simulink library "orocomplib"  (R2015b)
settings: Solver=ode45  StartTime=0.0  StopTime=10.0  RelTol=1e-3
settings Model: Creator=laurent  LastModifiedBy=admin
settings DataIOCC: SaveFormat=Array  SaveOutput=off  SignalLogging=off  DSMLogging=off  SaveTime=off
settings OptimizationCC: ExpressionDepthLimit=2147483647
settings DebuggingCC: UnderspecifiedInitializationDetection=Classic  MergeDetectMultiDrivingBlocksExec=none  SolverPrmCheckMsg=warning  StateNameClashWarn=warning
settings HardwareCC: ProdBitPerPointer=32  ProdLargestAtomicFloat=None  ProdIntDivRoundTo=Undefined  ProdEndianess=Unspecified  ProdWordSize=32  ProdHWDeviceType=32-bit Generic
settings GRTTargetCC: GeneratePreprocessorConditionals=Disable all
settings ConfigComp: CovModelRefEnable=Off

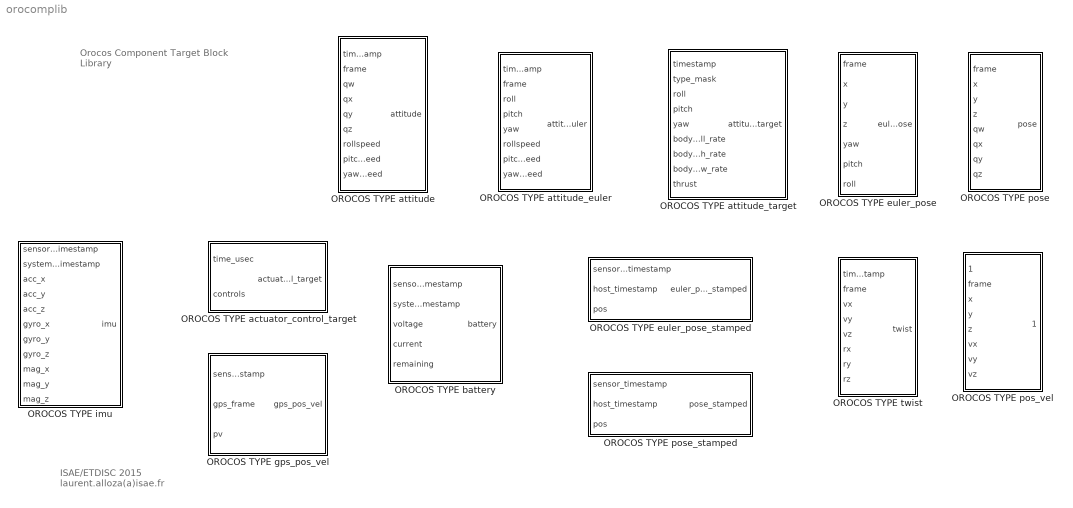
== system orocomplib ==
  note: ISAE/ETDISC 2015
      | laurent.alloza(a)isae.fr
  note: Orocos Component Target
      | Block Library
  OROCOS TYPE battery : Subsystem  InitFcn=|  mask(OROCOS TYPE battery){}
      | if not(exist('battery','var')),
      | load orotypes_isae;
      | end
      mask help: Creates an Orocos Port compatible type.
      settings: MinAlgLoopOccurrences=on  RTWSystemCode=Inline
  OROCOS TYPE imu : Subsystem  InitFcn=|  mask(OROCOS TYPE imu){}
      | if not(exist('imu','var')),
      | load orotypes_isae;
      | end
      mask help: Creates an Orocos Port compatible type.
      settings: MinAlgLoopOccurrences=on  RTWSystemCode=Inline
  OROCOS TYPE actuator_control_target : Subsystem  InitFcn=|  mask(OROCOS TYPE actuator_control_target){}
      | if not(exist('actuator_control_target','var')),
      | load orotypes_isae;
      | end
      mask help: Creates an Orocos Port compatible type.
      settings: MinAlgLoopOccurrences=on  RTWSystemCode=Inline
  OROCOS TYPE attitude : Subsystem  InitFcn=|  mask(OROCOS TYPE attitude){}
      | if not(exist('attitude','var')),
      | load orotypes_isae;
      | end
      mask help: Creates an Orocos Port compatible type.
      settings: MinAlgLoopOccurrences=on  RTWSystemCode=Inline
  OROCOS TYPE attitude_euler : Subsystem  InitFcn=|  mask(OROCOS TYPE attitude_euler){}
      | if not(exist('attitude_euler','var')),
      | load orotypes_isae;
      | end
      mask help: Creates an Orocos Port compatible type.
      settings: MinAlgLoopOccurrences=on  RTWSystemCode=Inline
  OROCOS TYPE attitude_target : Subsystem  InitFcn=|  mask(OROCOS TYPE attitude_target){}
      | if not(exist('attitude_target','var')),
      | load orotypes_isae;
      | end
      mask help: Creates an Orocos Port compatible type.
      settings: MinAlgLoopOccurrences=on  RTWSystemCode=Inline
  OROCOS TYPE euler_pose : Subsystem  InitFcn=|  mask(OROCOS TYPE euler_pose){}
      | if not(exist('euler_pose','var')),
      | load orotypes_isae;
      | end
      mask help: Creates an Orocos Port compatible type.
      settings: MinAlgLoopOccurrences=on  RTWSystemCode=Inline
  OROCOS TYPE euler_pose_stamped : Subsystem  InitFcn=|  mask(OROCOS TYPE euler_pose_stamped){}
      | if not(exist('euler_pose_stamped','var')),
      | load orotypes_isae;
      | end
      mask help: Creates an Orocos Port compatible type.
      settings: MinAlgLoopOccurrences=on  RTWSystemCode=Inline
  OROCOS TYPE gps_pos_vel : Subsystem  InitFcn=|  mask(OROCOS TYPE gps_pos_vel){}
      | if not(exist('gps_pos_vel','var')),
      | load orotypes_isae;
      | end
      mask help: Creates an Orocos Port compatible type.
      settings: MinAlgLoopOccurrences=on  RTWSystemCode=Inline
  OROCOS TYPE pos_vel : Subsystem  InitFcn=|  mask(OROCOS TYPE pos_vel){}
      | if not(exist('pos_vel','var')),
      | load orotypes_isae;
      | end
      mask help: Creates an Orocos Port compatible type.
      settings: MinAlgLoopOccurrences=on  RTWSystemCode=Inline
  OROCOS TYPE pose : Subsystem  InitFcn=|  mask(OROCOS TYPE pose){}
      | if not(exist('pose','var')),
      | load orotypes_isae;
      | end
      mask help: Creates an Orocos Port compatible type.
      settings: MinAlgLoopOccurrences=on  RTWSystemCode=Inline
  OROCOS TYPE pose_stamped : Subsystem  InitFcn=|  mask(OROCOS TYPE pose_stamped){}
      | if not(exist('pose_stamped','var')),
      | load orotypes_isae;
      | end
      mask help: Creates an Orocos Port compatible type.
      settings: MinAlgLoopOccurrences=on  RTWSystemCode=Inline
  OROCOS TYPE twist : Subsystem  InitFcn=|  mask(OROCOS TYPE twist){}
      | if not(exist('twist','var')),
      | load orotypes_isae;
      | end
      mask help: Creates an Orocos Port compatible type.
      settings: MinAlgLoopOccurrences=on  RTWSystemCode=Inline

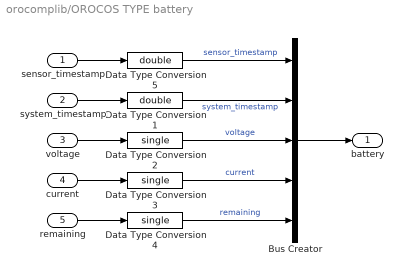
== system orocomplib/OROCOS TYPE battery ==
  sensor_timestamp : Inport  PortDimensions=1
  system_timestamp : Inport  Port=2  PortDimensions=1
  voltage : Inport  Port=3  PortDimensions=1
  current : Inport  Port=4  PortDimensions=1
  remaining : Inport  Port=5  PortDimensions=1
  Bus Creator : BusCreator  Inputs='sensor_timestamp','system_timestamp','voltage','current','remaining'  OutDataTypeStr=Bus: battery  NonVirtualBus=on
  Data Type Conversion1 : DataTypeConversion  OutDataTypeStr=double  RndMeth=Zero  LockScale=on
  Data Type Conversion2 : DataTypeConversion  OutDataTypeStr=single  RndMeth=Zero  LockScale=on
  Data Type Conversion3 : DataTypeConversion  OutDataTypeStr=single  RndMeth=Zero  LockScale=on
  Data Type Conversion4 : DataTypeConversion  OutDataTypeStr=single  RndMeth=Zero  LockScale=on
  Data Type Conversion5 : DataTypeConversion  OutDataTypeStr=double  RndMeth=Zero  LockScale=on
  battery : Outport
  wires:
  system_timestamp/1 -> Data Type Conversion1/1
  Data Type Conversion1/1 -> Bus Creator/2  "system_timestamp"
  Data Type Conversion4/1 -> Bus Creator/5  "remaining"
  remaining/1 -> Data Type Conversion4/1
  Data Type Conversion3/1 -> Bus Creator/4  "current"
  current/1 -> Data Type Conversion3/1
  Data Type Conversion2/1 -> Bus Creator/3  "voltage"
  voltage/1 -> Data Type Conversion2/1
  sensor_timestamp/1 -> Data Type Conversion5/1
  Bus Creator/1 -> battery/1
  Data Type Conversion5/1 -> Bus Creator/1  "sensor_timestamp"

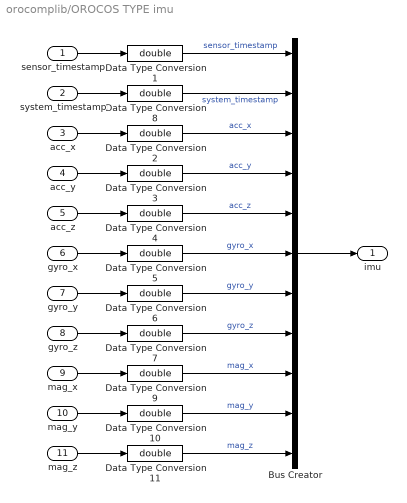
== system orocomplib/OROCOS TYPE imu ==
  sensor_timestamp : Inport  PortDimensions=1
  system_timestamp : Inport  Port=2  PortDimensions=1
  acc_x : Inport  Port=3  PortDimensions=1
  acc_y : Inport  Port=4  PortDimensions=1
  acc_z : Inport  Port=5  PortDimensions=1
  gyro_x : Inport  Port=6  PortDimensions=1
  gyro_y : Inport  Port=7  PortDimensions=1
  gyro_z : Inport  Port=8  PortDimensions=1
  mag_x : Inport  Port=9  PortDimensions=1
  mag_y : Inport  Port=10  PortDimensions=1
  mag_z : Inport  Port=11  PortDimensions=1
  Bus Creator : BusCreator  Inputs=11  OutDataTypeStr=Bus: imu  NonVirtualBus=on
  Data Type Conversion{1..11} (11 alike) : DataTypeConversion  OutDataTypeStr=double  RndMeth=Zero  LockScale=on
  imu : Outport
  wires:
  system_timestamp/1 -> Data Type Conversion8/1
  Data Type Conversion8/1 -> Bus Creator/2  "system_timestamp"
  Data Type Conversion2/1 -> Bus Creator/3  "acc_x"
  acc_x/1 -> Data Type Conversion2/1
  sensor_timestamp/1 -> Data Type Conversion1/1
  Bus Creator/1 -> imu/1
  Data Type Conversion1/1 -> Bus Creator/1  "sensor_timestamp"
  Data Type Conversion3/1 -> Bus Creator/4  "acc_y"
  acc_y/1 -> Data Type Conversion3/1
  Data Type Conversion4/1 -> Bus Creator/5  "acc_z"
  acc_z/1 -> Data Type Conversion4/1
  Data Type Conversion5/1 -> Bus Creator/6  "gyro_x"
  gyro_x/1 -> Data Type Conversion5/1
  Data Type Conversion6/1 -> Bus Creator/7  "gyro_y"
  gyro_y/1 -> Data Type Conversion6/1
  Data Type Conversion7/1 -> Bus Creator/8  "gyro_z"
  gyro_z/1 -> Data Type Conversion7/1
  Data Type Conversion9/1 -> Bus Creator/9  "mag_x"
  mag_x/1 -> Data Type Conversion9/1
  Data Type Conversion10/1 -> Bus Creator/10  "mag_y"
  mag_y/1 -> Data Type Conversion10/1
  Data Type Conversion11/1 -> Bus Creator/11  "mag_z"
  mag_z/1 -> Data Type Conversion11/1

== system orocomplib/OROCOS TYPE actuator_control_target ==
  time_usec : Inport  PortDimensions=1
  controls : Inport  Port=2  PortDimensions=8
  Bus Creator : BusCreator  Inputs=2  OutDataTypeStr=Bus: actuator_control_target  NonVirtualBus=on
  Data Type Conversion1 : DataTypeConversion  OutDataTypeStr=double  RndMeth=Zero  LockScale=on
  Data Type Conversion2 : DataTypeConversion  OutDataTypeStr=single  RndMeth=Zero  LockScale=on
  actuator_control_target : Outport
  wires:
  Data Type Conversion2/1 -> Bus Creator/2  "controls"
  controls/1 -> Data Type Conversion2/1
  time_usec/1 -> Data Type Conversion1/1
  Bus Creator/1 -> actuator_control_target/1
  Data Type Conversion1/1 -> Bus Creator/1  "time_usec"

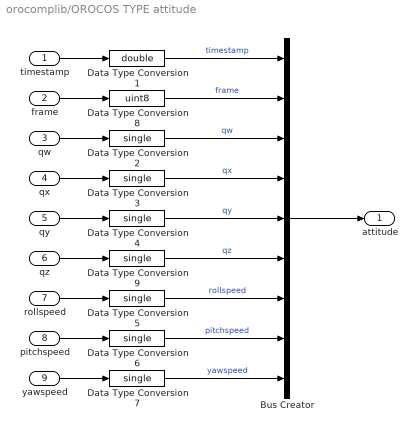
== system orocomplib/OROCOS TYPE attitude ==
  timestamp : Inport  PortDimensions=1
  frame : Inport  Port=2  PortDimensions=1
  qw : Inport  Port=3  PortDimensions=1
  qx : Inport  Port=4  PortDimensions=1
  qy : Inport  Port=5  PortDimensions=1
  qz : Inport  Port=6  PortDimensions=1
  rollspeed : Inport  Port=7  PortDimensions=1
  pitchspeed : Inport  Port=8  PortDimensions=1
  yawspeed : Inport  Port=9  PortDimensions=1
  Bus Creator : BusCreator  Inputs='timestamp','frame','qw','qx','qy','qz','rollspeed','pitchspeed','yawspeed'  OutDataTypeStr=Bus: attitude  NonVirtualBus=on
  Data Type Conversion1 : DataTypeConversion  OutDataTypeStr=double  RndMeth=Zero  LockScale=on
  Data Type Conversion{2..7,9} (7 alike) : DataTypeConversion  OutDataTypeStr=single  RndMeth=Zero  LockScale=on
  Data Type Conversion8 : DataTypeConversion  OutDataTypeStr=uint8  RndMeth=Zero  LockScale=on
  attitude : Outport
  wires:
  qz/1 -> Data Type Conversion9/1
  Data Type Conversion9/1 -> Bus Creator/6  "qz"
  Data Type Conversion1/1 -> Bus Creator/1  "timestamp"
  frame/1 -> Data Type Conversion8/1
  Bus Creator/1 -> attitude/1
  timestamp/1 -> Data Type Conversion1/1
  qw/1 -> Data Type Conversion2/1
  Data Type Conversion2/1 -> Bus Creator/3  "qw"
  qx/1 -> Data Type Conversion3/1
  Data Type Conversion3/1 -> Bus Creator/4  "qx"
  qy/1 -> Data Type Conversion4/1
  Data Type Conversion4/1 -> Bus Creator/5  "qy"
  rollspeed/1 -> Data Type Conversion5/1
  pitchspeed/1 -> Data Type Conversion6/1
  yawspeed/1 -> Data Type Conversion7/1
  Data Type Conversion5/1 -> Bus Creator/7  "rollspeed"
  Data Type Conversion6/1 -> Bus Creator/8  "pitchspeed"
  Data Type Conversion7/1 -> Bus Creator/9  "yawspeed"
  Data Type Conversion8/1 -> Bus Creator/2  "frame"

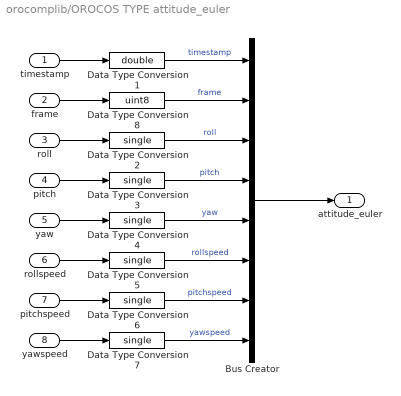
== system orocomplib/OROCOS TYPE attitude_euler ==
  timestamp : Inport  PortDimensions=1
  frame : Inport  Port=2  PortDimensions=1
  roll : Inport  Port=3  PortDimensions=1
  pitch : Inport  Port=4  PortDimensions=1
  yaw : Inport  Port=5  PortDimensions=1
  rollspeed : Inport  Port=6  PortDimensions=1
  pitchspeed : Inport  Port=7  PortDimensions=1
  yawspeed : Inport  Port=8  PortDimensions=1
  Bus Creator : BusCreator  Inputs=8  OutDataTypeStr=Bus: attitude_euler  NonVirtualBus=on
  Data Type Conversion1 : DataTypeConversion  OutDataTypeStr=double  RndMeth=Zero  LockScale=on
  Data Type Conversion{2..7} (6 alike) : DataTypeConversion  OutDataTypeStr=single  RndMeth=Zero  LockScale=on
  Data Type Conversion8 : DataTypeConversion  OutDataTypeStr=uint8  RndMeth=Zero  LockScale=on
  attitude_euler : Outport
  wires:
  Data Type Conversion1/1 -> Bus Creator/1  "timestamp"
  frame/1 -> Data Type Conversion8/1
  Bus Creator/1 -> attitude_euler/1
  timestamp/1 -> Data Type Conversion1/1
  roll/1 -> Data Type Conversion2/1
  Data Type Conversion2/1 -> Bus Creator/3  "roll"
  pitch/1 -> Data Type Conversion3/1
  Data Type Conversion3/1 -> Bus Creator/4  "pitch"
  yaw/1 -> Data Type Conversion4/1
  Data Type Conversion4/1 -> Bus Creator/5  "yaw"
  rollspeed/1 -> Data Type Conversion5/1
  pitchspeed/1 -> Data Type Conversion6/1
  yawspeed/1 -> Data Type Conversion7/1
  Data Type Conversion5/1 -> Bus Creator/6  "rollspeed"
  Data Type Conversion6/1 -> Bus Creator/7  "pitchspeed"
  Data Type Conversion7/1 -> Bus Creator/8  "yawspeed"
  Data Type Conversion8/1 -> Bus Creator/2  "frame"

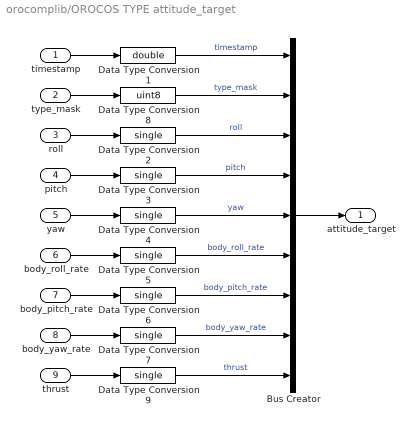
== system orocomplib/OROCOS TYPE attitude_target ==
  timestamp : Inport  PortDimensions=1
  type_mask : Inport  Port=2  PortDimensions=1
  roll : Inport  Port=3  PortDimensions=1
  pitch : Inport  Port=4  PortDimensions=1
  yaw : Inport  Port=5  PortDimensions=1
  body_roll_rate : Inport  Port=6  PortDimensions=1
  body_pitch_rate : Inport  Port=7  PortDimensions=1
  body_yaw_rate : Inport  Port=8  PortDimensions=1
  thrust : Inport  Port=9  PortDimensions=1
  Bus Creator : BusCreator  Inputs='timestamp','type_mask','roll','pitch','yaw','body_roll_rate','body_pitch_rate','body_yaw_rate','thrust'  OutDataTypeStr=Bus: attitude_target  NonVirtualBus=on
  Data Type Conversion1 : DataTypeConversion  OutDataTypeStr=double  RndMeth=Zero  LockScale=on
  Data Type Conversion{2..7,9} (7 alike) : DataTypeConversion  OutDataTypeStr=single  RndMeth=Zero  LockScale=on
  Data Type Conversion8 : DataTypeConversion  OutDataTypeStr=uint8  RndMeth=Zero  LockScale=on
  attitude_target : Outport
  wires:
  Data Type Conversion1/1 -> Bus Creator/1  "timestamp"
  type_mask/1 -> Data Type Conversion8/1
  Bus Creator/1 -> attitude_target/1
  timestamp/1 -> Data Type Conversion1/1
  roll/1 -> Data Type Conversion2/1
  Data Type Conversion2/1 -> Bus Creator/3  "roll"
  pitch/1 -> Data Type Conversion3/1
  Data Type Conversion3/1 -> Bus Creator/4  "pitch"
  yaw/1 -> Data Type Conversion4/1
  Data Type Conversion4/1 -> Bus Creator/5  "yaw"
  body_roll_rate/1 -> Data Type Conversion5/1
  body_pitch_rate/1 -> Data Type Conversion6/1
  body_yaw_rate/1 -> Data Type Conversion7/1
  Data Type Conversion5/1 -> Bus Creator/6  "body_roll_rate"
  Data Type Conversion6/1 -> Bus Creator/7  "body_pitch_rate"
  Data Type Conversion7/1 -> Bus Creator/8  "body_yaw_rate"
  Data Type Conversion8/1 -> Bus Creator/2  "type_mask"
  thrust/1 -> Data Type Conversion9/1
  Data Type Conversion9/1 -> Bus Creator/9  "thrust"

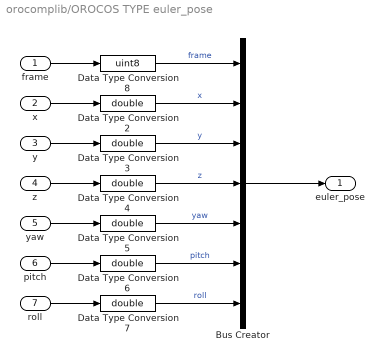
== system orocomplib/OROCOS TYPE euler_pose ==
  frame : Inport  PortDimensions=1
  x : Inport  Port=2  PortDimensions=1
  y : Inport  Port=3  PortDimensions=1
  z : Inport  Port=4  PortDimensions=1
  yaw : Inport  Port=5  PortDimensions=1
  pitch : Inport  Port=6  PortDimensions=1
  roll : Inport  Port=7  PortDimensions=1
  Bus Creator : BusCreator  Inputs='frame','x','y','z','yaw','pitch','roll'  OutDataTypeStr=Bus: euler_pose  NonVirtualBus=on
  Data Type Conversion{2..7} (6 alike) : DataTypeConversion  OutDataTypeStr=double  RndMeth=Zero  LockScale=on
  Data Type Conversion8 : DataTypeConversion  OutDataTypeStr=uint8  RndMeth=Zero  LockScale=on
  euler_pose : Outport
  wires:
  frame/1 -> Data Type Conversion8/1
  Bus Creator/1 -> euler_pose/1
  x/1 -> Data Type Conversion2/1
  Data Type Conversion2/1 -> Bus Creator/2  "x"
  y/1 -> Data Type Conversion3/1
  Data Type Conversion3/1 -> Bus Creator/3  "y"
  z/1 -> Data Type Conversion4/1
  Data Type Conversion4/1 -> Bus Creator/4  "z"
  yaw/1 -> Data Type Conversion5/1
  pitch/1 -> Data Type Conversion6/1
  roll/1 -> Data Type Conversion7/1
  Data Type Conversion5/1 -> Bus Creator/5  "yaw"
  Data Type Conversion6/1 -> Bus Creator/6  "pitch"
  Data Type Conversion7/1 -> Bus Creator/7  "roll"
  Data Type Conversion8/1 -> Bus Creator/1  "frame"

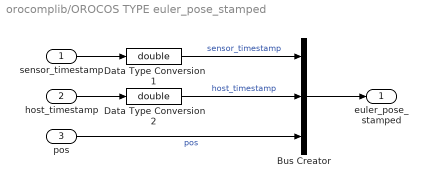
== system orocomplib/OROCOS TYPE euler_pose_stamped ==
  sensor_timestamp : Inport  PortDimensions=1
  host_timestamp : Inport  Port=2  PortDimensions=1
  pos : Inport  Port=3  OutDataTypeStr=Bus: euler_pose  PortDimensions=1  LockScale=on
  Bus Creator : BusCreator  Inputs='sensor_timestamp','host_timestamp','pos'  OutDataTypeStr=Bus: euler_pose_stamped  NonVirtualBus=on
  Data Type Conversion1 : DataTypeConversion  OutDataTypeStr=double  RndMeth=Zero  LockScale=on
  Data Type Conversion2 : DataTypeConversion  OutDataTypeStr=double  RndMeth=Zero  LockScale=on
  euler_pose_stamped : Outport
  wires:
  Data Type Conversion1/1 -> Bus Creator/1  "sensor_timestamp"
  host_timestamp/1 -> Data Type Conversion2/1
  Bus Creator/1 -> euler_pose_stamped/1
  sensor_timestamp/1 -> Data Type Conversion1/1
  pos/1 -> Bus Creator/3  "pos"
  Data Type Conversion2/1 -> Bus Creator/2  "host_timestamp"

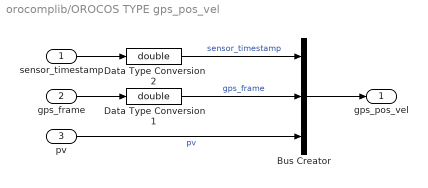
== system orocomplib/OROCOS TYPE gps_pos_vel ==
  sensor_timestamp : Inport  PortDimensions=1
  gps_frame : Inport  Port=2  PortDimensions=1
  pv : Inport  Port=3  OutDataTypeStr=Bus: pos_vel  PortDimensions=1  LockScale=on
  Bus Creator : BusCreator  Inputs='sensor_timestamp','gps_frame','pv'  OutDataTypeStr=Bus: gps_pos_vel  NonVirtualBus=on
  Data Type Conversion1 : DataTypeConversion  OutDataTypeStr=double  RndMeth=Zero  LockScale=on
  Data Type Conversion2 : DataTypeConversion  OutDataTypeStr=double  RndMeth=Zero  LockScale=on
  gps_pos_vel : Outport
  wires:
  Data Type Conversion1/1 -> Bus Creator/2  "gps_frame"
  pv/1 -> Bus Creator/3  "pv"
  sensor_timestamp/1 -> Data Type Conversion2/1
  Bus Creator/1 -> gps_pos_vel/1
  gps_frame/1 -> Data Type Conversion1/1
  Data Type Conversion2/1 -> Bus Creator/1  "sensor_timestamp"

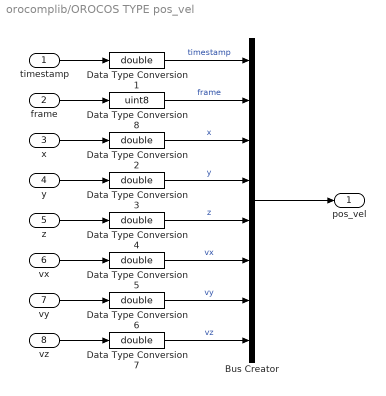
== system orocomplib/OROCOS TYPE pos_vel ==
  timestamp : Inport  PortDimensions=1
  frame : Inport  Port=2  PortDimensions=1
  x : Inport  Port=3  PortDimensions=1
  y : Inport  Port=4  PortDimensions=1
  z : Inport  Port=5  PortDimensions=1
  vx : Inport  Port=6  PortDimensions=1
  vy : Inport  Port=7  PortDimensions=1
  vz : Inport  Port=8  PortDimensions=1
  Bus Creator : BusCreator  Inputs='timestamp','frame','x','y','z','vx','vy','vz'  OutDataTypeStr=Bus: pos_vel  NonVirtualBus=on
  Data Type Conversion{1..7} (7 alike) : DataTypeConversion  OutDataTypeStr=double  RndMeth=Zero  LockScale=on
  Data Type Conversion8 : DataTypeConversion  OutDataTypeStr=uint8  RndMeth=Zero  LockScale=on
  pos_vel : Outport
  wires:
  Data Type Conversion1/1 -> Bus Creator/1  "timestamp"
  frame/1 -> Data Type Conversion8/1
  Bus Creator/1 -> pos_vel/1
  timestamp/1 -> Data Type Conversion1/1
  x/1 -> Data Type Conversion2/1
  Data Type Conversion2/1 -> Bus Creator/3  "x"
  y/1 -> Data Type Conversion3/1
  Data Type Conversion3/1 -> Bus Creator/4  "y"
  z/1 -> Data Type Conversion4/1
  Data Type Conversion4/1 -> Bus Creator/5  "z"
  vx/1 -> Data Type Conversion5/1
  vy/1 -> Data Type Conversion6/1
  vz/1 -> Data Type Conversion7/1
  Data Type Conversion5/1 -> Bus Creator/6  "vx"
  Data Type Conversion6/1 -> Bus Creator/7  "vy"
  Data Type Conversion7/1 -> Bus Creator/8  "vz"
  Data Type Conversion8/1 -> Bus Creator/2  "frame"

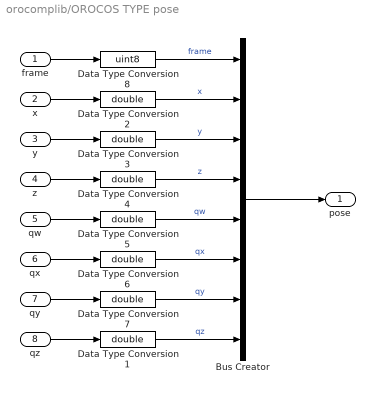
== system orocomplib/OROCOS TYPE pose ==
  frame : Inport  PortDimensions=1
  x : Inport  Port=2  PortDimensions=1
  y : Inport  Port=3  PortDimensions=1
  z : Inport  Port=4  PortDimensions=1
  qw : Inport  Port=5  PortDimensions=1
  qx : Inport  Port=6  PortDimensions=1
  qy : Inport  Port=7  PortDimensions=1
  qz : Inport  Port=8  PortDimensions=1
  Bus Creator : BusCreator  Inputs='frame','x','y','z','qw','qx','qy','qz'  OutDataTypeStr=Bus: pose  NonVirtualBus=on
  Data Type Conversion{1..7} (7 alike) : DataTypeConversion  OutDataTypeStr=double  RndMeth=Zero  LockScale=on
  Data Type Conversion8 : DataTypeConversion  OutDataTypeStr=uint8  RndMeth=Zero  LockScale=on
  pose : Outport
  wires:
  Data Type Conversion1/1 -> Bus Creator/8  "qz"
  qz/1 -> Data Type Conversion1/1
  Data Type Conversion8/1 -> Bus Creator/1  "frame"
  Data Type Conversion7/1 -> Bus Creator/7  "qy"
  Data Type Conversion6/1 -> Bus Creator/6  "qx"
  Data Type Conversion5/1 -> Bus Creator/5  "qw"
  qy/1 -> Data Type Conversion7/1
  qx/1 -> Data Type Conversion6/1
  qw/1 -> Data Type Conversion5/1
  Data Type Conversion4/1 -> Bus Creator/4  "z"
  z/1 -> Data Type Conversion4/1
  Data Type Conversion3/1 -> Bus Creator/3  "y"
  y/1 -> Data Type Conversion3/1
  Data Type Conversion2/1 -> Bus Creator/2  "x"
  x/1 -> Data Type Conversion2/1
  Bus Creator/1 -> pose/1
  frame/1 -> Data Type Conversion8/1

== system orocomplib/OROCOS TYPE pose_stamped ==
  sensor_timestamp : Inport  PortDimensions=1
  host_timestamp : Inport  Port=2  PortDimensions=1
  pos : Inport  Port=3  OutDataTypeStr=Bus: pose  PortDimensions=1  LockScale=on
  Bus Creator : BusCreator  Inputs='sensor_timestamp','host_timestamp','pos'  OutDataTypeStr=Bus: pose_stamped  NonVirtualBus=on
  Data Type Conversion1 : DataTypeConversion  OutDataTypeStr=double  RndMeth=Zero  LockScale=on
  Data Type Conversion2 : DataTypeConversion  OutDataTypeStr=double  RndMeth=Zero  LockScale=on
  pose_stamped : Outport
  wires:
  Data Type Conversion1/1 -> Bus Creator/2  "host_timestamp"
  pos/1 -> Bus Creator/3  "pos"
  sensor_timestamp/1 -> Data Type Conversion2/1
  Bus Creator/1 -> pose_stamped/1
  host_timestamp/1 -> Data Type Conversion1/1
  Data Type Conversion2/1 -> Bus Creator/1  "sensor_timestamp"

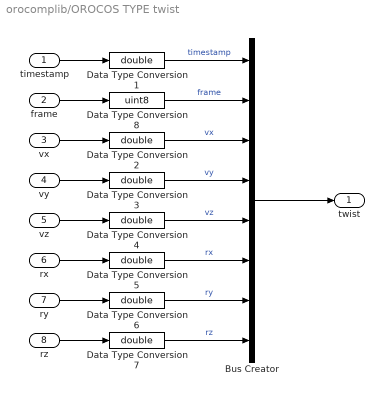
== system orocomplib/OROCOS TYPE twist ==
  timestamp : Inport  PortDimensions=1
  frame : Inport  Port=2  PortDimensions=1
  vx : Inport  Port=3  PortDimensions=1
  vy : Inport  Port=4  PortDimensions=1
  vz : Inport  Port=5  PortDimensions=1
  rx : Inport  Port=6  PortDimensions=1
  ry : Inport  Port=7  PortDimensions=1
  rz : Inport  Port=8  PortDimensions=1
  Bus Creator : BusCreator  Inputs='timestamp','frame','vx','vy','vz','rx','ry','rz'  OutDataTypeStr=Bus: twist  NonVirtualBus=on
  Data Type Conversion{1..7} (7 alike) : DataTypeConversion  OutDataTypeStr=double  RndMeth=Zero  LockScale=on
  Data Type Conversion8 : DataTypeConversion  OutDataTypeStr=uint8  RndMeth=Zero  LockScale=on
  twist : Outport
  wires:
  Data Type Conversion8/1 -> Bus Creator/2  "frame"
  Data Type Conversion7/1 -> Bus Creator/8  "rz"
  Data Type Conversion6/1 -> Bus Creator/7  "ry"
  Data Type Conversion5/1 -> Bus Creator/6  "rx"
  rz/1 -> Data Type Conversion7/1
  ry/1 -> Data Type Conversion6/1
  rx/1 -> Data Type Conversion5/1
  Data Type Conversion4/1 -> Bus Creator/5  "vz"
  vz/1 -> Data Type Conversion4/1
  Data Type Conversion3/1 -> Bus Creator/4  "vy"
  vy/1 -> Data Type Conversion3/1
  Data Type Conversion2/1 -> Bus Creator/3  "vx"
  vx/1 -> Data Type Conversion2/1
  timestamp/1 -> Data Type Conversion1/1
  Bus Creator/1 -> twist/1
  frame/1 -> Data Type Conversion8/1
  Data Type Conversion1/1 -> Bus Creator/1  "timestamp"
